simulink model "case1"  (R2023a)
settings: Solver=VariableStepAuto  StartTime=0.0  StopTime=30.0  RelTol=1e-3
undefined symbols (not defined in the file): fdesignblkfcn, gcbh
libraries: dspfdesign x4, vrlib x1
settings Model: Creator=elsibo  LastModifiedBy=roumaissa
settings OptimizationCC: ReuseModelBlockBuffer=off
settings DebuggingCC: UnconnectedInputMsg=warning  UnconnectedOutputMsg=warning  UnconnectedLineMsg=warning
settings ModelReferenceCC: EnableRefExpFcnMdlSchedulingChecks=on
settings RTWCC: DLArmComputeVersion=19.05

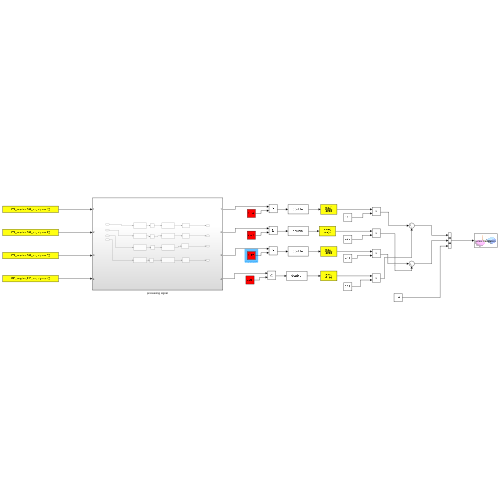
[thumbnail: Simulink's stored preview of the top-level diagram]
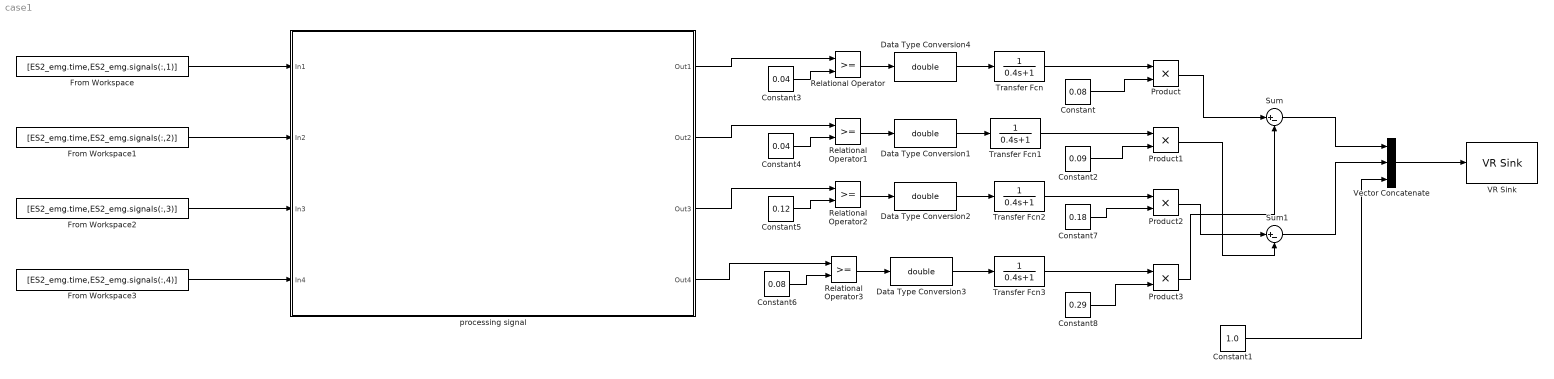
== system case1 ==
  Constant : Constant  Value=0.08
  Constant1 : Constant  Value=1.0
  Constant2 : Constant  Value=0.09
  Constant3 : Constant  Value=0.04
  Constant4 : Constant  Value=0.04
  Constant5 : Constant  Value=0.12
  Constant6 : Constant  Value=0.08
  Constant7 : Constant  Value=0.18
  Constant8 : Constant  Value=0.29
  Data Type Conversion{1..4} (4 alike) : DataTypeConversion  OutMin=[0.2]  OutMax=[1000]  OutDataTypeStr=double  SaturateOnIntegerOverflow=off  RndMeth=Floor
  From Workspace : FromWorkspace  VariableName=[ES2_emg.time,ES2_emg.signals(:,1)]  SampleTime=1/1000
  From Workspace1 : FromWorkspace  VariableName=[ES2_emg.time,ES2_emg.signals(:,2)]  SampleTime=1/1000
  From Workspace2 : FromWorkspace  VariableName=[ES2_emg.time,ES2_emg.signals(:,3)]  SampleTime=1/1000
  From Workspace3 : FromWorkspace  VariableName=[ES2_emg.time,ES2_emg.signals(:,4)]  SampleTime=1/1000
  Product{,1..3} (4 alike) : Product
  Relational Operator{,1..3} (4 alike) : RelationalOperator  OutDataTypeStr=boolean  RndMeth=Simplest  InputSameDT=off
  Sum : Sum  Inputs=|+-
  Sum1 : Sum  Inputs=|+-
  Transfer Fcn{,1..3} (4 alike) : TransferFcn  Denominator=[0.4 1]
  VR Sink : vrlib/VR Sink  InstantiateOnLoad=on  SampleTime=0.1  ViewEnable=on  RemoteChange=off  RemoteView=off  FieldsWritten=cursor.translation.3.1.1.double  WorldFileName=8_palline_color.wrl  AutoView=off  VideoDimensions=[]  AllowVariableSize=off
  Vector Concatenate : Concatenate  NumInputs=3
  processing signal : Subsystem
  wires:
  Constant3/1 -> Relational Operator/2
  Relational Operator/1 -> Data Type Conversion4/1
  Relational Operator1/1 -> Data Type Conversion1/1
  Constant4/1 -> Relational Operator1/2
  Relational Operator2/1 -> Data Type Conversion2/1
  Constant5/1 -> Relational Operator2/2
  Relational Operator3/1 -> Data Type Conversion3/1
  Constant6/1 -> Relational Operator3/2
  Data Type Conversion3/1 -> Transfer Fcn3/1
  Data Type Conversion2/1 -> Transfer Fcn2/1
  Data Type Conversion1/1 -> Transfer Fcn1/1
  Data Type Conversion4/1 -> Transfer Fcn/1
  Transfer Fcn1/1 -> Product1/1
  Transfer Fcn2/1 -> Product2/1
  Transfer Fcn3/1 -> Product3/1
  Product/1 -> Sum/1
  Product2/1 -> Sum1/1
  Sum/1 -> Vector Concatenate/1
  Sum1/1 -> Vector Concatenate/2
  Constant1/1 -> Vector Concatenate/3
  Vector Concatenate/1 -> VR Sink/1
  Product3/1 -> Sum/2
  Product1/1 -> Sum1/2
  From Workspace3/1 -> processing signal/4(In4)
  From Workspace2/1 -> processing signal/3(In3)
  From Workspace1/1 -> processing signal/2(In2)
  From Workspace/1 -> processing signal/1(In1)
  processing signal/1(Out1) -> Relational Operator/1
  processing signal/2(Out2) -> Relational Operator1/1
  processing signal/3(Out3) -> Relational Operator2/1
  processing signal/4(Out4) -> Relational Operator3/1
  Transfer Fcn/1 -> Product/1
  Constant/1 -> Product/2
  Constant2/1 -> Product1/2
  Constant7/1 -> Product2/2
  Constant8/1 -> Product3/2

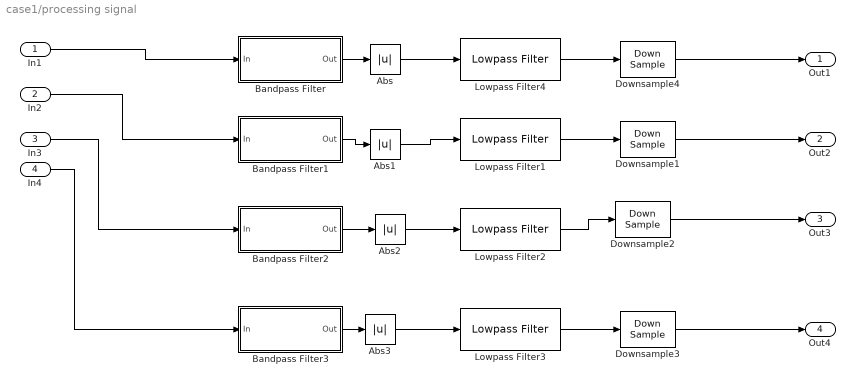
== system case1/processing signal ==
  In1 : Inport
  In2 : Inport  Port=2
  In3 : Inport  Port=3
  In4 : Inport  Port=4
  Abs{,1..3} (4 alike) : Abs  SaturateOnIntegerOverflow=off
  Bandpass Filter : Subsystem  DialogController=fdesignblkfcn  InitFcn=fdesignblkfcn(gcbh, {'InitFcn'});  mask(Bandpass Filter){}
      mask help: Design a bandpass filter
      settings: CopyFcn=fdesignblkfcn(gcbh, {'CopyFcn'});
      mask Help: helpview(mapfilelocation('dsp'), 'dspbandpassfilter');
      mask Display: disp('Bandpass');
  Bandpass Filter1 : Subsystem  DialogController=fdesignblkfcn  InitFcn=fdesignblkfcn(gcbh, {'InitFcn'});  mask(Bandpass Filter){}
      mask help: Design a bandpass filter
      settings: CopyFcn=fdesignblkfcn(gcbh, {'CopyFcn'});
      mask Help: helpview(mapfilelocation('dsp'), 'dspbandpassfilter');
      mask Display: disp('Bandpass');
  Bandpass Filter2 : Subsystem  DialogController=fdesignblkfcn  InitFcn=fdesignblkfcn(gcbh, {'InitFcn'});  mask(Bandpass Filter){}
      mask help: Design a bandpass filter
      settings: CopyFcn=fdesignblkfcn(gcbh, {'CopyFcn'});
      mask Help: helpview(mapfilelocation('dsp'), 'dspbandpassfilter');
      mask Display: disp('Bandpass');
  Bandpass Filter3 : Subsystem  DialogController=fdesignblkfcn  InitFcn=fdesignblkfcn(gcbh, {'InitFcn'});  mask(Bandpass Filter){}
      mask help: Design a bandpass filter
      settings: CopyFcn=fdesignblkfcn(gcbh, {'CopyFcn'});
      mask Help: helpview(mapfilelocation('dsp'), 'dspbandpassfilter');
      mask Display: disp('Bandpass');
  Downsample{1..4} (4 alike) : DownSample  N=100  RateOptions=Allow multirate processing
  Lowpass Filter{1..4} (4 alike) : dspfdesign/Lowpass Filter  FilterType=FIR  DesignForMinimumOrder=on  FilterOrder=50  PassbandFrequency=1e3  StopbandFrequency=5e3  PassbandRipple=0.1  StopbandAttenuation=80  SampleRateMode=Specify on dialog  SampleRate=44100  SimulateUsing=Interpreted execution  roundingMode=Floor  coeffsDataTypeStr=fixdt(1,16)
  Out1 : Outport
  Out2 : Outport  Port=2
  Out3 : Outport  Port=3
  Out4 : Outport  Port=4
  wires:
  Bandpass Filter1/1(Out) -> Abs1/1
  Abs1/1 -> Lowpass Filter1/1
  Bandpass Filter3/1(Out) -> Abs3/1
  Bandpass Filter/1(Out) -> Abs/1
  Abs/1 -> Lowpass Filter4/1
  Bandpass Filter2/1(Out) -> Abs2/1
  Abs2/1 -> Lowpass Filter2/1
  Abs3/1 -> Lowpass Filter3/1
  Lowpass Filter2/1 -> Downsample2/1
  Lowpass Filter3/1 -> Downsample3/1
  Lowpass Filter1/1 -> Downsample1/1
  Lowpass Filter4/1 -> Downsample4/1
  In1/1 -> Bandpass Filter/1(In)
  In2/1 -> Bandpass Filter1/1(In)
  In3/1 -> Bandpass Filter2/1(In)
  In4/1 -> Bandpass Filter3/1(In)
  Downsample1/1 -> Out2/1
  Downsample4/1 -> Out1/1
  Downsample2/1 -> Out3/1
  Downsample3/1 -> Out4/1

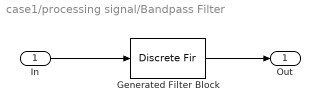
== system case1/processing signal/Bandpass Filter ==
  In : Inport
  Generated Filter Block : DiscreteFir  Tag=BlockMethodSubSystem  Coefficients=[0.0858980048566166249 0.0520786279754757025 -0.0994053436914434235 0.0135831519514875414 -0.0538866276248172876 0.00387436549081726384 -0.028401820868103278 0.00254018756536164092 -0.0104438154349616504 0.0024745447461073781 0.00401687504188876464 0.00235138339428692892 0.0153358382804895353 0.00309905498380235291 0.0226439192297243561 0.00584913788288324125 0.0251768114891905807 0.0110810472179320892 0.023027830667927341 0.0181002991305211844 0.0175130800707560576 0.0250386900455970215 0.0107549207084791966 0.0294778815550422457 0.00505958386037309252 0.0291499572930629738 0.00231750847441022966 0.0227233532183568968 0.00320765883427242497 0.0104612349040572247 0.00671392201303706512 -0.00561396203127093648 0.0102558775940295565 -0.0219812639834285582 0.0103879546700692688 -0.0345352141556959508 0.00395681818876779477 -0.0398775820234136547 -0.0110238072701888054 -0.0361350674372840144 -0.0347821929209543301 -0.0235894563232318007 -0.064962129429258525 -0.00499593179626695374 -0.0969031197365728958 0.0154172518528037789 -0.12536697763726562 0.0328234804291783963 -0.145037688666316195 0.042569528484803644 0.847893838599677263 0.042569528484803644 -0.145037688666316195 0.0328234804291783963 -0.12536697763726562 0.0154172518528037789 -0.0969031197365728958 -0.00499593179626695374 -0.064962129429258525 -0.0235894563232318007 -0.0347821929209543301 -0.0361350674372840144 -0.0110238072701888054 -0.0398775820234136547 0.00395681818876779477 -0.0345352141556959508 0.0103879546700692688 -0.0219812639834285582 0.0102558775940295565 -0.00561396203127093648 0.00671392201303706512 0.0104612349040572247 0.00320765883427242497 0.0227233532183568968 0.00231750847441022966 0.0291499572930629738 0.00505958386037309252 0.0294778815550422457 0.0107549207084791966 0.0250386900455970215 0.0175130800707560576 0.0181002991305211844 0.023027830667927341 0.0110810472179320892 0.0251768114891905807 0.00584913788288324125 0.0226439192297243561 0.00309905498380235291 0.0153358382804895353 0.00235138339428692892 0.00401687504188876464 0.0024745447461073781 -0.0104438154349616504 0.00254018756536164092 -0.028401820868103278 0.00387436549081726384 -0.0538866276248172876 0.0135831519514875414 -0.0994053436914434235 0.0520786279754757025 0.0858980048566166249]  InputProcessing=Columns as channels (frame based)
  Out : Outport  VectorParamsAs1DForOutWhenUnconnected=off
  wires:
  In/1 -> Generated Filter Block/1
  Generated Filter Block/1 -> Out/1

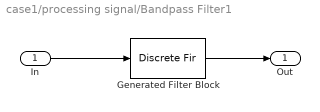
== system case1/processing signal/Bandpass Filter1 ==
  In : Inport
  Generated Filter Block : DiscreteFir  Tag=BlockMethodSubSystem  Coefficients=[0.0858980048566166249 0.0520786279754757025 -0.0994053436914434235 0.0135831519514875414 -0.0538866276248172876 0.00387436549081726384 -0.028401820868103278 0.00254018756536164092 -0.0104438154349616504 0.0024745447461073781 0.00401687504188876464 0.00235138339428692892 0.0153358382804895353 0.00309905498380235291 0.0226439192297243561 0.00584913788288324125 0.0251768114891905807 0.0110810472179320892 0.023027830667927341 0.0181002991305211844 0.0175130800707560576 0.0250386900455970215 0.0107549207084791966 0.0294778815550422457 0.00505958386037309252 0.0291499572930629738 0.00231750847441022966 0.0227233532183568968 0.00320765883427242497 0.0104612349040572247 0.00671392201303706512 -0.00561396203127093648 0.0102558775940295565 -0.0219812639834285582 0.0103879546700692688 -0.0345352141556959508 0.00395681818876779477 -0.0398775820234136547 -0.0110238072701888054 -0.0361350674372840144 -0.0347821929209543301 -0.0235894563232318007 -0.064962129429258525 -0.00499593179626695374 -0.0969031197365728958 0.0154172518528037789 -0.12536697763726562 0.0328234804291783963 -0.145037688666316195 0.042569528484803644 0.847893838599677263 0.042569528484803644 -0.145037688666316195 0.0328234804291783963 -0.12536697763726562 0.0154172518528037789 -0.0969031197365728958 -0.00499593179626695374 -0.064962129429258525 -0.0235894563232318007 -0.0347821929209543301 -0.0361350674372840144 -0.0110238072701888054 -0.0398775820234136547 0.00395681818876779477 -0.0345352141556959508 0.0103879546700692688 -0.0219812639834285582 0.0102558775940295565 -0.00561396203127093648 0.00671392201303706512 0.0104612349040572247 0.00320765883427242497 0.0227233532183568968 0.00231750847441022966 0.0291499572930629738 0.00505958386037309252 0.0294778815550422457 0.0107549207084791966 0.0250386900455970215 0.0175130800707560576 0.0181002991305211844 0.023027830667927341 0.0110810472179320892 0.0251768114891905807 0.00584913788288324125 0.0226439192297243561 0.00309905498380235291 0.0153358382804895353 0.00235138339428692892 0.00401687504188876464 0.0024745447461073781 -0.0104438154349616504 0.00254018756536164092 -0.028401820868103278 0.00387436549081726384 -0.0538866276248172876 0.0135831519514875414 -0.0994053436914434235 0.0520786279754757025 0.0858980048566166249]  InputProcessing=Columns as channels (frame based)
  Out : Outport  VectorParamsAs1DForOutWhenUnconnected=off
  wires:
  In/1 -> Generated Filter Block/1
  Generated Filter Block/1 -> Out/1

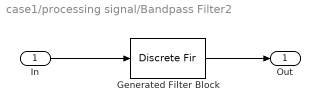
== system case1/processing signal/Bandpass Filter2 ==
  In : Inport
  Generated Filter Block : DiscreteFir  Tag=BlockMethodSubSystem  Coefficients=[0.0858980048566166249 0.0520786279754757025 -0.0994053436914434235 0.0135831519514875414 -0.0538866276248172876 0.00387436549081726384 -0.028401820868103278 0.00254018756536164092 -0.0104438154349616504 0.0024745447461073781 0.00401687504188876464 0.00235138339428692892 0.0153358382804895353 0.00309905498380235291 0.0226439192297243561 0.00584913788288324125 0.0251768114891905807 0.0110810472179320892 0.023027830667927341 0.0181002991305211844 0.0175130800707560576 0.0250386900455970215 0.0107549207084791966 0.0294778815550422457 0.00505958386037309252 0.0291499572930629738 0.00231750847441022966 0.0227233532183568968 0.00320765883427242497 0.0104612349040572247 0.00671392201303706512 -0.00561396203127093648 0.0102558775940295565 -0.0219812639834285582 0.0103879546700692688 -0.0345352141556959508 0.00395681818876779477 -0.0398775820234136547 -0.0110238072701888054 -0.0361350674372840144 -0.0347821929209543301 -0.0235894563232318007 -0.064962129429258525 -0.00499593179626695374 -0.0969031197365728958 0.0154172518528037789 -0.12536697763726562 0.0328234804291783963 -0.145037688666316195 0.042569528484803644 0.847893838599677263 0.042569528484803644 -0.145037688666316195 0.0328234804291783963 -0.12536697763726562 0.0154172518528037789 -0.0969031197365728958 -0.00499593179626695374 -0.064962129429258525 -0.0235894563232318007 -0.0347821929209543301 -0.0361350674372840144 -0.0110238072701888054 -0.0398775820234136547 0.00395681818876779477 -0.0345352141556959508 0.0103879546700692688 -0.0219812639834285582 0.0102558775940295565 -0.00561396203127093648 0.00671392201303706512 0.0104612349040572247 0.00320765883427242497 0.0227233532183568968 0.00231750847441022966 0.0291499572930629738 0.00505958386037309252 0.0294778815550422457 0.0107549207084791966 0.0250386900455970215 0.0175130800707560576 0.0181002991305211844 0.023027830667927341 0.0110810472179320892 0.0251768114891905807 0.00584913788288324125 0.0226439192297243561 0.00309905498380235291 0.0153358382804895353 0.00235138339428692892 0.00401687504188876464 0.0024745447461073781 -0.0104438154349616504 0.00254018756536164092 -0.028401820868103278 0.00387436549081726384 -0.0538866276248172876 0.0135831519514875414 -0.0994053436914434235 0.0520786279754757025 0.0858980048566166249]  InputProcessing=Columns as channels (frame based)
  Out : Outport  VectorParamsAs1DForOutWhenUnconnected=off
  wires:
  In/1 -> Generated Filter Block/1
  Generated Filter Block/1 -> Out/1

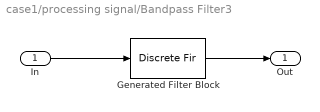
== system case1/processing signal/Bandpass Filter3 ==
  In : Inport
  Generated Filter Block : DiscreteFir  Tag=BlockMethodSubSystem  Coefficients=[0.0858980048566166249 0.0520786279754757025 -0.0994053436914434235 0.0135831519514875414 -0.0538866276248172876 0.00387436549081726384 -0.028401820868103278 0.00254018756536164092 -0.0104438154349616504 0.0024745447461073781 0.00401687504188876464 0.00235138339428692892 0.0153358382804895353 0.00309905498380235291 0.0226439192297243561 0.00584913788288324125 0.0251768114891905807 0.0110810472179320892 0.023027830667927341 0.0181002991305211844 0.0175130800707560576 0.0250386900455970215 0.0107549207084791966 0.0294778815550422457 0.00505958386037309252 0.0291499572930629738 0.00231750847441022966 0.0227233532183568968 0.00320765883427242497 0.0104612349040572247 0.00671392201303706512 -0.00561396203127093648 0.0102558775940295565 -0.0219812639834285582 0.0103879546700692688 -0.0345352141556959508 0.00395681818876779477 -0.0398775820234136547 -0.0110238072701888054 -0.0361350674372840144 -0.0347821929209543301 -0.0235894563232318007 -0.064962129429258525 -0.00499593179626695374 -0.0969031197365728958 0.0154172518528037789 -0.12536697763726562 0.0328234804291783963 -0.145037688666316195 0.042569528484803644 0.847893838599677263 0.042569528484803644 -0.145037688666316195 0.0328234804291783963 -0.12536697763726562 0.0154172518528037789 -0.0969031197365728958 -0.00499593179626695374 -0.064962129429258525 -0.0235894563232318007 -0.0347821929209543301 -0.0361350674372840144 -0.0110238072701888054 -0.0398775820234136547 0.00395681818876779477 -0.0345352141556959508 0.0103879546700692688 -0.0219812639834285582 0.0102558775940295565 -0.00561396203127093648 0.00671392201303706512 0.0104612349040572247 0.00320765883427242497 0.0227233532183568968 0.00231750847441022966 0.0291499572930629738 0.00505958386037309252 0.0294778815550422457 0.0107549207084791966 0.0250386900455970215 0.0175130800707560576 0.0181002991305211844 0.023027830667927341 0.0110810472179320892 0.0251768114891905807 0.00584913788288324125 0.0226439192297243561 0.00309905498380235291 0.0153358382804895353 0.00235138339428692892 0.00401687504188876464 0.0024745447461073781 -0.0104438154349616504 0.00254018756536164092 -0.028401820868103278 0.00387436549081726384 -0.0538866276248172876 0.0135831519514875414 -0.0994053436914434235 0.0520786279754757025 0.0858980048566166249]  InputProcessing=Columns as channels (frame based)
  Out : Outport  VectorParamsAs1DForOutWhenUnconnected=off
  wires:
  In/1 -> Generated Filter Block/1
  Generated Filter Block/1 -> Out/1
